simulink model "Problem1"  (R2020b)
settings: Solver=VariableStepAuto  StartTime=0.0  StopTime=100  MaxStep=0.01  RelTol=1e-3
model workspace (MAT data in the model file):
  K1 = Simulink.Parameter
  K1.Value = 50
  K1.DataType = 'auto'
  K1.Dimensions = [1 1]
  M1 = Simulink.Parameter
  M1.Value = 100
  M1.DataType = 'auto'
  M1.Dimensions = [1 1]
  M2 = Simulink.Parameter
  M2.Value = 70
  M2.DataType = 'auto'
  M2.Dimensions = [1 1]
  b = Simulink.Parameter
  b.Value = 50
  b.DataType = 'auto'
  b.Dimensions = [1 1]
  k12 = Simulink.Parameter
  k12.Value = 30
  k12.DataType = 'auto'
  k12.Dimensions = [1 1]
settings Model: OrderedModelArguments=off  Creator=hp  LastModifiedBy=hp

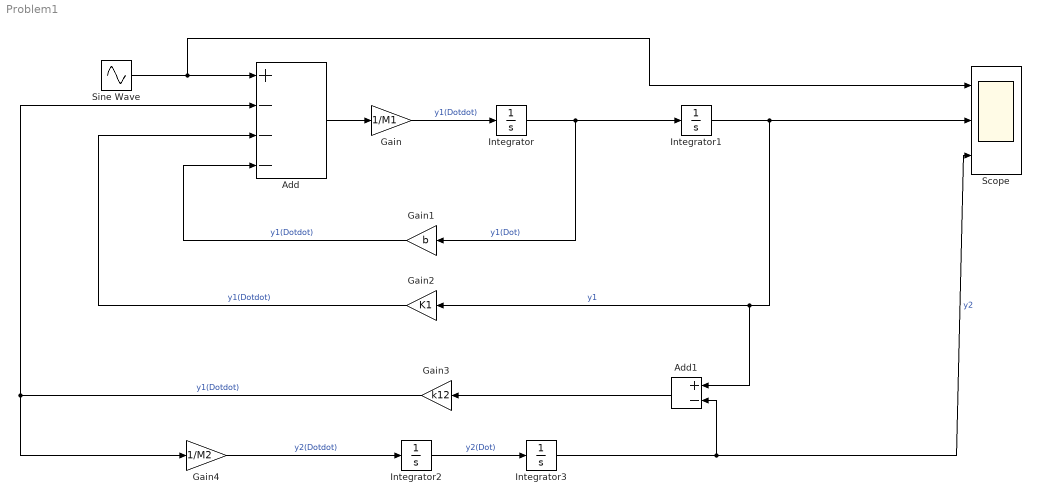
== system Problem1 ==
  Add : Sum  Inputs=+---
  Add1 : Sum  Inputs=+-
  Gain : Gain  Gain=1/M1
  Gain1 : Gain  Gain=b
  Gain2 : Gain  Gain=K1
  Gain3 : Gain  Gain=k12  mask{Parameter1=80.0}
      mask prompts: Parameter1 "K12"
  Gain4 : Gain  Gain=1/M2
  Integrator : Integrator  InitialCondition=1
  Integrator1 : Integrator
  Integrator2 : Integrator
  Integrator3 : Integrator
  Scope : Scope  NumInputPorts=3
  Sine Wave : Sin  Amplitude=2  Frequency=2*pi*10  SampleTime=0.005
  wires:
  Sine Wave/1 -> Scope/1, Add/1
  Add/1 -> Gain/1
  Integrator/1 -> Gain1/1, Integrator1/1  "y1(Dot)"
  Integrator1/1 -> Add1/1, Gain2/1, Scope/2  "y1"
  Gain/1 -> Integrator/1  "y1(Dotdot)"
  Gain1/1 -> Add/4  "y1(Dotdot)"
  Gain2/1 -> Add/3  "y1(Dotdot)"
  Add1/1 -> Gain3/1
  Gain3/1 -> Gain4/1, Add/2  "y1(Dotdot)"
  Gain4/1 -> Integrator2/1  "y2(Dotdot)"
  Integrator2/1 -> Integrator3/1  "y2(Dot)"
  Integrator3/1 -> Add1/2, Scope/3  "y2"
